simulink model "Ejercicio_3_DB_Caso_1"  (R2023a)
settings: Solver=VariableStepAuto  StartTime=0.0  StopTime=2  RelTol=1e-6  EnableMultiTasking=on
values from neighbouring files (symbols this model uses):
  Ap = [-Ra/La 0 0 -Kb*A2/(La*R*A1) ... (first row only)    [Ejercicio_1.m]    (also in Ejercicio_2y3.m = [0 1 0)
  Bp = [A/La 0 0 0]'    [Ejercicio_1.m]    (also in Ejercicio_2y3.m = [0 0 1]')
  Cp = [0 0 1/km 0]    [Ejercicio_1.m]    (also in Ejercicio_2y3.m = [b0 0 0])
  Dp = 0    [Ejercicio_1.m]    (also in Ejercicio_2y3.m)
  g0 = y_inf/(Cp*inv(Bp*Ke-Ap)*Bp)    [Ejercicio_2y3.m]
  Ke = acker(Ap,Bp,P_LC)    [Ejercicio_2y3.m]
  Kest = acker(Ap',Cp',P_Est)'    [Ejercicio_2y3.m]
settings Model: Creator=54115  LastModifiedBy=franc
settings SolverCC: AlgebraicLoopSolver=TrustRegion
settings DataIOCC: ReturnWorkspaceOutputs=off
settings OptimizationCC: LifeSpan=inf
settings DebuggingCC: UnconnectedInputMsg=warning  UnconnectedOutputMsg=warning  UnconnectedLineMsg=warning  SFUnexpectedBacktrackingDiag=warning  SFNoUnconditionalDefaultTransitionDiag=warning  ArithmeticOperatorsInVariantConditions=warning
settings ModelReferenceCC: EnableRefExpFcnMdlSchedulingChecks=on
settings SFSimCC: SimUseLocalCustomCode=off  CustomCodeUndefinedFunction=UseInterfaceOnly
settings RTWCC: RTWUseLocalCustomCode=off
settings CodeAppCC: StateflowObjectComments=on
settings GRTTargetCC: TargetLangStandard=C89/C90 (ANSI)
settings ConfigComp: CovMetricSettings=dw  CovSaveCumulativeToWorkspaceVar=on  CovSaveSingleToWorkspaceVar=on  CovExternalEMLEnable=off

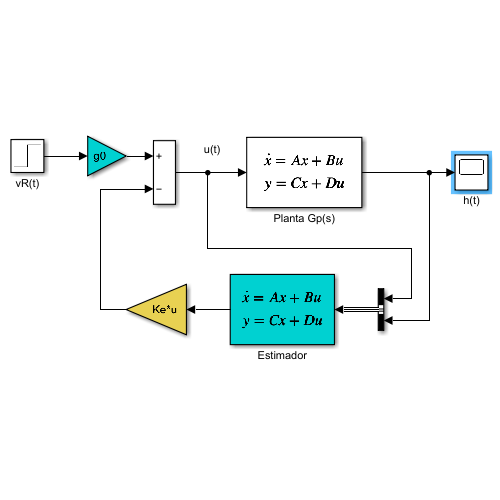
[thumbnail: Simulink's stored preview of the top-level diagram]
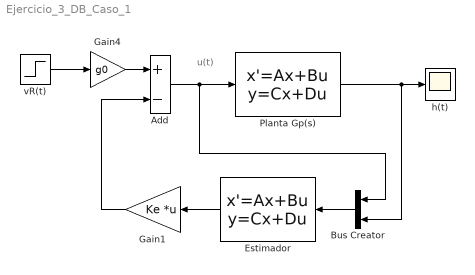
== system Ejercicio_3_DB_Caso_1 ==
  note: u(t)
  Add : Sum  Inputs=+-
  Bus Creator : BusCreator  Inputs=2
  Estimador : StateSpace  A=Ap - Kest*Cp  B=[Bp Kest]  C=eye(3)  D=[0 0;0 0;0 0]  InitialCondition=0
  Gain1 : Gain  Gain=Ke  Multiplication=Matrix(K*u)
  Gain4 : Gain  Gain=g0
  Planta Gp(s) : StateSpace  A=Ap  B=Bp  C=Cp  D=Dp  InitialCondition=0
  h(t) : Scope
  vR(t) : Step  Time=0  SampleTime=0
  wires:
  Add/1 -> Bus Creator/1, Planta Gp(s)/1
  vR(t)/1 -> Gain4/1
  Planta Gp(s)/1 -> h(t)/1, Bus Creator/2
  Gain4/1 -> Add/1
  Bus Creator/1 -> Estimador/1
  Estimador/1 -> Gain1/1
  Gain1/1 -> Add/2
